simulink model "BandPassFilter_td0200ka"  (R2015a)
settings: Solver=ode23t  StartTime=0.0  StopTime=2  RelTol=1e-3
libraries: fl_lib x15, nesl_utility x5, powerlib x3
settings Model: Creator=saifur  LastModifiedBy=saifur

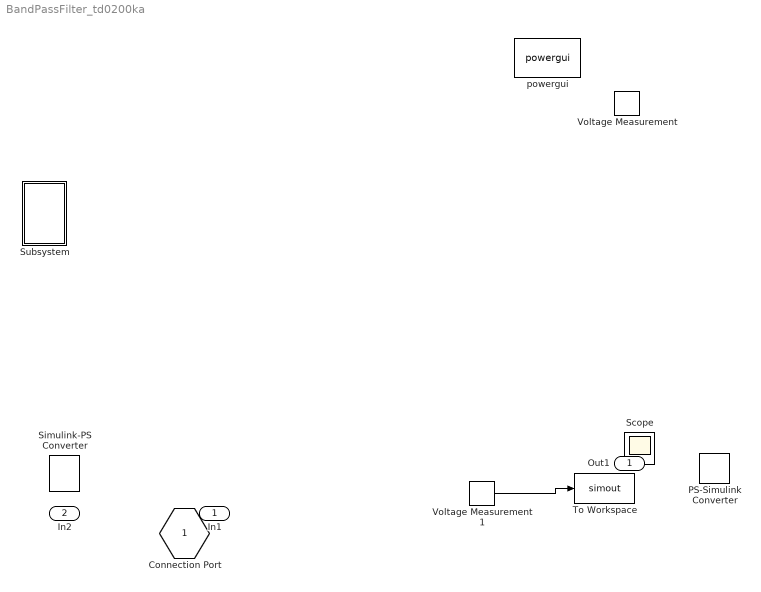
== system BandPassFilter_td0200ka ==
  In1 : Inport
  In2 : Inport  Port=2
  PS-Simulink Converter : nesl_utility/PS-Simulink Converter  PhysicalDomain=network_engine_domain  SubClassName=ps_output  LeftPortType=input  RightPortType=output  PseudoPeriodic=off  Frequencies=[]  Unit=1  AffineConversion=off
  Scope : Scope
  Simulink-PS Converter : nesl_utility/Simulink-PS Converter  PhysicalDomain=network_engine_domain  SubClassName=ps_input  LeftPortType=input  RightPortType=output  PseudoPeriodic=off  Frequencies=[]  NoiseDistribution=none  NoiseParameters=[]  Unit=1  AffineConversion=off  InputFiltering=off  SimscapeFilterOrder=1  InputFilterTimeConstant=0.001  UdotUserProvided=1
  Subsystem : Subsystem
  To Workspace : ToWorkspace  VariableName=simout  SaveFormat=Timeseries  SampleTime=-1
  Voltage Measurement : powerlib/Measurements/Voltage Measurement  PhasorSimulation=off  OutputType=Complex  PSBequivalent=0
  Voltage Measurement1 : powerlib/Measurements/Voltage Measurement  PhasorSimulation=off  OutputType=Complex  PSBequivalent=0
  powergui : powerlib/powergui  Priority=1  SimulationMode=Discrete  SolverType=Tustin/Backward Euler (TBE)  SampleTime=50e-6  frequency=60  SPID=off  DisableSnubberDevices=off  DisableRonSwitches=off  DisableVfSwitches=off  SwTol=0  DisplayEquations=off  Interpol=off  methode=off  Ts=100  FunctionMessages=off  echomessages=off  HookPort=off  EnableUseOfTLC=off  x0status=blocks  frequencyindice=60  Pbase=100e6  ErrMax=1e-4  Iterations=50  UnitsV=kV  UnitsW=MW  buscounter=0  RestoreLinks=warning  ResistiveCurrentMeasurement=off  Frange=[0:2:500]  Ylog=off  Xlog=on  ShowGrid=off  save=off  variable=ZData  structure=0  ZoomFFT=off  StartTime=0.0  cycles=1  DisplayStyle=1  fundamental=60  FreqAxis=off  MaxFrequency=1000  frequencyindicesteady=1  RmsSteady=1  display=off
  Connection Port : PMIOPort  Port=1  Side=Left
  Out1 : Outport
  wires:
  Voltage Measurement1/1 -> To Workspace/1

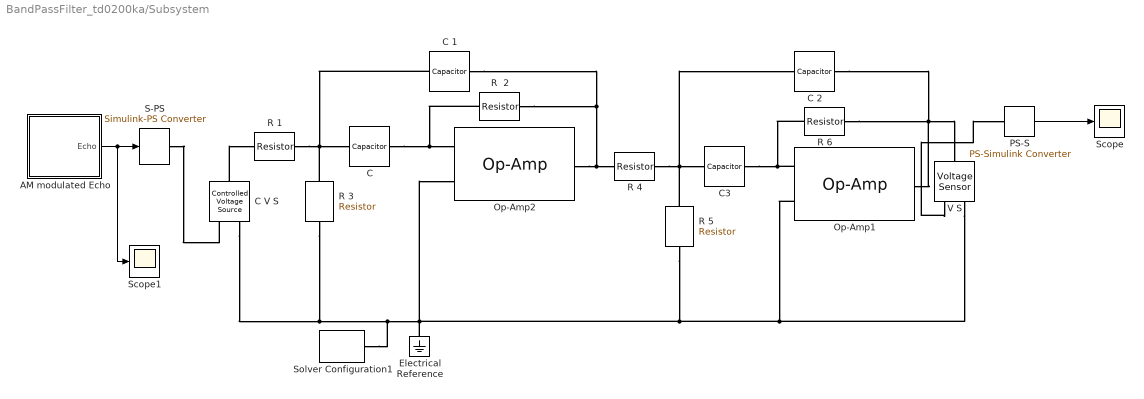
== system BandPassFilter_td0200ka/Subsystem ==
  AM modulated Echo : Subsystem
  C : fl_lib/Electrical/Electrical Elements/Capacitor  c=10 nF  r=1e-6 Ohm  g=0 1/Ohm  i_specify=off  i_priority=High  i=0 A  v_specify=off  v_priority=High  v=0 V  vc_specify=off  vc_priority=High  vc=0 V
  "C 1 " : fl_lib/Electrical/Electrical Elements/Capacitor  c=1e-6 F  r=1e-6 Ohm  g=0 1/Ohm  i_specify=off  i_priority=High  i=0 A  v_specify=off  v_priority=High  v=0 V  vc_specify=off  vc_priority=High  vc=0 V
  C 2 : fl_lib/Electrical/Electrical Elements/Capacitor  c=1e-6 F  r=1e-6 Ohm  g=0 1/Ohm  i_specify=off  i_priority=High  i=0 A  v_specify=off  v_priority=High  v=0 V  vc_specify=off  vc_priority=High  vc=0 V
  C V S : fl_lib/Electrical/Electrical Sources/Controlled Voltage Source
  C3 : fl_lib/Electrical/Electrical Elements/Capacitor  c=10 nF  r=1e-6 Ohm  g=0 1/Ohm  i_specify=off  i_priority=High  i=0 A  v_specify=off  v_priority=High  v=0 V  vc_specify=off  vc_priority=High  vc=0 V
  Electrical Reference : fl_lib/Electrical/Electrical Elements/Electrical Reference
  Op-Amp1 : fl_lib/Electrical/Electrical Elements/Op-Amp  outI_specify=off  outI_priority=High  outI=0 A
  Op-Amp2 : fl_lib/Electrical/Electrical Elements/Op-Amp  outI_specify=off  outI_priority=High  outI=0 A
  PS-S : nesl_utility/PS-Simulink Converter  PhysicalDomain=network_engine_domain  SubClassName=ps_output  LeftPortType=input  RightPortType=output  PseudoPeriodic=off  Frequencies=[]  Unit=1  AffineConversion=off
  R  2 : fl_lib/Electrical/Electrical Elements/Resistor  R=4.73 kOhm  i_specify=off  i_priority=High  i=0 A  v_specify=off  v_priority=High  v=0 V
  R 1 : fl_lib/Electrical/Electrical Elements/Resistor  R=519.8 Ohm  i_specify=off  i_priority=High  i=0 A  v_specify=off  v_priority=High  v=0 V
  R 3 : fl_lib/Electrical/Electrical Elements/Resistor  R=0.91 Ohm  i_specify=off  i_priority=High  i=0 A  v_specify=off  v_priority=High  v=0 V
  R 4 : fl_lib/Electrical/Electrical Elements/Resistor  R=763.73 Ohm  i_specify=off  i_priority=High  i=0 A  v_specify=off  v_priority=High  v=0 V
  R 5 : fl_lib/Electrical/Electrical Elements/Resistor  R=1.34 kOhm  i_specify=off  i_priority=High  i=0 A  v_specify=off  v_priority=High  v=0 V
  R 6 : fl_lib/Electrical/Electrical Elements/Resistor  R=6.95 kOhm  i_specify=off  i_priority=High  i=0 A  v_specify=off  v_priority=High  v=0 V
  S-PS : nesl_utility/Simulink-PS Converter  PhysicalDomain=network_engine_domain  SubClassName=ps_input  LeftPortType=input  RightPortType=output  PseudoPeriodic=off  Frequencies=[]  NoiseDistribution=none  NoiseParameters=[]  Unit=V  AffineConversion=off  InputFiltering=off  SimscapeFilterOrder=1  InputFilterTimeConstant=0.001  UdotUserProvided=1
  Scope : Scope
      settings: YMin=-0.045  YMax=0.045
  Scope1 : Scope
      settings: YMin=-8e-05  YMax=8e-05  SaveName=ScopeData2
  Solver Configuration1 : nesl_utility/Solver Configuration  PhysicalDomain=network_engine_domain  SubClassName=solver  LeftPortType=input  RightPortType=generic  Accelerate=off  Tones=[]  Harmonics=[]  SimulateNoise=off  Profile=off  UseLocalSampling=off  EnableSwitchedLinearOptims=on  FrequencyDomain=off  UseCCode=off  RelTol=0.001  AbsTol=1e-06  MinStep=1e-09  ToWorkspace=off  RevertToSquareIcSolve=off  NumHomotopyIterations=100  DoDC=on  ResidualTolerance=1e-09  UseLocalSolver=off  LocalSolverChoice=NE_BACKWARD_EULER_ADVANCER  LocalSolverSampleTime=0.001  DoFixedCost=off  MaxNonlinIter=3  MaxModeIter=2  LinearAlgebra=Sparse  DelaysMemoryBudget=1024  AutomaticFiltering=on  FilteringTimeConstant=0.001
  V S : fl_lib/Electrical/Electrical Sensors/Voltage Sensor
  wires:
  AM modulated Echo/1(Echo) -> Scope1/1, S-PS/1
  PS-S/1 -> Scope/1
  connections:
  C V S/LConn1 -- R 1/RConn1
  C/RConn1 -- R  2/RConn1 -- Op-Amp2/LConn2
  C3/RConn1 -- Op-Amp1/LConn1 -- R 6/LConn1
  C 2/RConn1 -- Op-Amp1/RConn1 -- V S/LConn1 -- R 6/RConn1
  Op-Amp2/RConn1 -- R  2/LConn1 -- "C 1 "/RConn1 -- R 4/LConn1
  R 1/LConn1 -- C/LConn1 -- "C 1 "/LConn1 -- R 3/LConn1
  Electrical Reference/LConn1 -- C V S/RConn2 -- R 3/RConn1 -- Solver Configuration1/RConn1 -- Op-Amp2/LConn1 -- Op-Amp1/LConn2 -- V S/RConn2 -- R 5/RConn1
  R 4/RConn1 -- C3/LConn1 -- C 2/LConn1 -- R 5/LConn1
  S-PS/RConn1 -- C V S/RConn1
  V S/RConn1 -- PS-S/LConn1

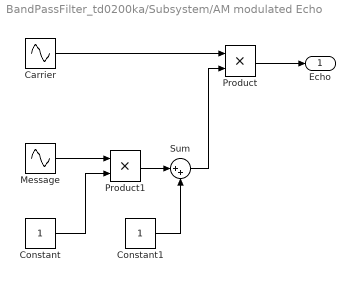
== system BandPassFilter_td0200ka/Subsystem/AM modulated Echo ==
  Carrier : Sin  Amplitude=50  Frequency=2*pi*100  SampleTime=1/5000
  Constant : Constant
  Constant1 : Constant
  Message : Sin  Amplitude=50  Frequency=2*pi*2  Phase=2  SampleTime=1/5000
  Product : Product
  Product1 : Product
  Sum : Sum  Inputs=|++
  Echo : Outport
  wires:
  Product/1 -> Echo/1
  Message/1 -> Product1/1
  Carrier/1 -> Product/1
  Constant/1 -> Product1/2
  Constant1/1 -> Sum/2
  Sum/1 -> Product/2
  Product1/1 -> Sum/1
